simulink model "Paper2_4Spline"  (R2014a)
settings: Solver=ode45  StartTime=0.0  StopTime=2.37  RelTol=1e-3
settings Model: Creator=Think127  LastModifiedBy=Think127

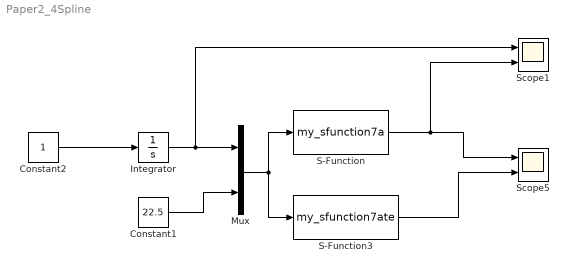
== system Paper2_4Spline ==
  Constant1 : Constant  Value=22.5
  Constant2 : Constant
  Integrator : Integrator  LimitOutput=on  LowerSaturationLimit=0
  Mux : Mux  Inputs=2
  S-Function : S-Function  FunctionName=my_sfunction7a  EnableBusSupport=off
  S-Function3 : S-Function  FunctionName=my_sfunction7ate  EnableBusSupport=off
  Scope1 : Scope  NumInputPorts=2
      settings: YMin=7.5~600  YMax=9.75~1800
  Scope5 : Scope  NumInputPorts=2
      settings: YMin=7.5~600  YMax=9.75~1800  SaveName=ScopeData7
  wires:
  Mux/1 -> S-Function3/1, S-Function/1
  Constant1/1 -> Mux/2
  Constant2/1 -> Integrator/1
  Integrator/1 -> Scope1/1, Mux/1
  S-Function/1 -> Scope1/2, Scope5/1
  S-Function3/1 -> Scope5/2
